simulink model "double_integrator"  (R2013a)
settings: Solver=ode45  StartTime=0.0  StopTime=100  RelTol=1e-3
InitFcn:
  | param
undefined symbols (not defined in the file or in its folder): AP, ctrl, P
libraries: simulink x1
settings Model: Creator=beard  LastModifiedBy=beard

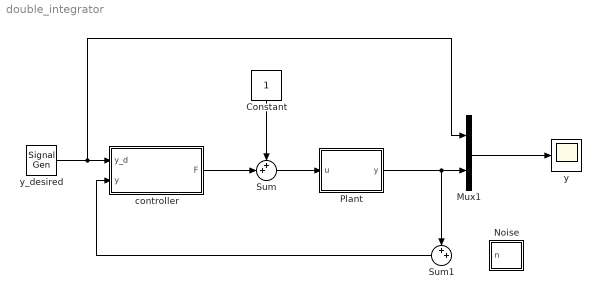
== system double_integrator ==
  Constant : Constant
  Mux1 : Mux  Inputs=2
  Noise : Subsystem
  Plant : Subsystem
  Sum : Sum  Inputs=++|
  Sum1 : Sum  Inputs=++|
  controller : Subsystem
  y : Scope
  y_desired : SignalGenerator  WaveForm=square  Frequency=0.02
  wires:
  controller/1(F) -> Sum/2
  Sum1/1 -> controller/2(y)
  Sum/1 -> Plant/1(u)
  Mux1/1 -> y/1
  y_desired/1 -> Mux1/1, controller/1(y_d)
  Plant/1(y) -> Sum1/1, Mux1/2
  Constant/1 -> Sum/1

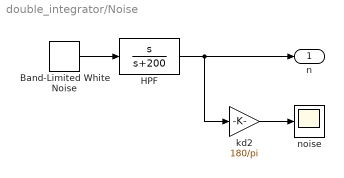
== system double_integrator/Noise ==
  Band-Limited White Noise : simulink/Sources/Band-Limited White Noise  Cov=[0.0001]  Ts=P.Ts  seed=[23341]
  HPF : TransferFcn  Numerator=[1 0]  Denominator=[1 200]
  kd2 : Gain  Gain=180/pi
  noise : Scope
      settings: YMin=-7  YMax=8  SaveName=ScopeData2
  n : Outport
  wires:
  Band-Limited White Noise/1 -> HPF/1
  kd2/1 -> noise/1
  HPF/1 -> kd2/1, n/1

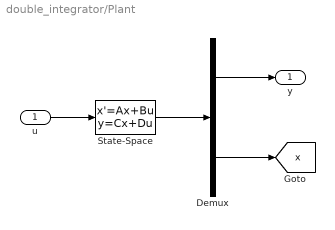
== system double_integrator/Plant ==
  u : Inport
  Demux : Demux  Outputs=[1;2]
  State-Space : StateSpace  A=AP.A  B=AP.B  C=[AP.C; eye(2)]  D=[P.D; 0; 0]  X0=[0;0]
  y : Outport
  tag scope: x=global
  wires:
  u/1 -> State-Space/1
  State-Space/1 -> Demux/1
  Demux/1 -> y/1
  Demux/2 -> [x]

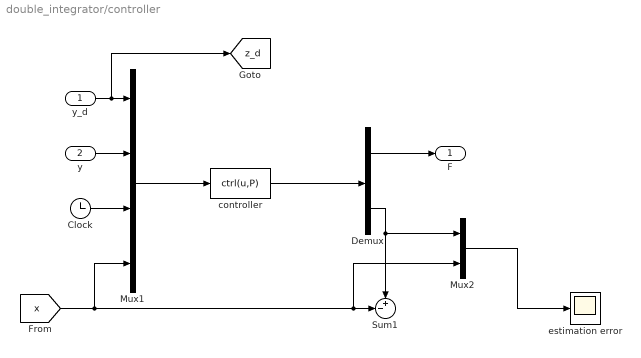
== system double_integrator/controller ==
  y_d : Inport
  y : Inport  Port=2
  Clock : Clock
  Demux : Demux  Outputs=[1;2]
  Mux1 : Mux
  Mux2 : Mux  Inputs=2
  Sum1 : Sum  Inputs=+-|
  controller : MATLABFcn  MATLABFcn=ctrl(u,P)  OutputDimensions=1+2  SampleTime=P.Ts
  estimation error : Scope
      settings: TimeRange=100  YMin=-8  YMax=7
  F : Outport
  tag scope: z_d=global
  wires:
  Clock/1 -> Mux1/3
  y/1 -> Mux1/2
  y_d/1 -> [z_d], Mux1/1
  Mux1/1 -> controller/1
  Demux/1 -> F/1
  controller/1 -> Demux/1
  [x] -> Mux1/4, Mux2/2, Sum1/2
  Demux/2 -> Mux2/1, Sum1/1
  Mux2/1 -> estimation error/1
